simulink model "testGaitGeneration"  (R2016b)
settings: Solver=FixedStepAuto  StartTime=0.0  StopTime=20  FixedStep=0.001  RelTol=1e-3
undefined symbols (not defined in the file or in its folder): angleHip, angleKnee, GaitGenerator, lookUpTable, sitDownHip, sitDownKnee, standUpHip, standUpKnee, stateMachineHandler, walkRWHip, walkRWKnee
libraries: VariousLibrary x5, simulink x1
settings Model: DataDictionary=ModelDictionary.sldd  Creator=Taeke  LastModifiedBy=lucadelaat

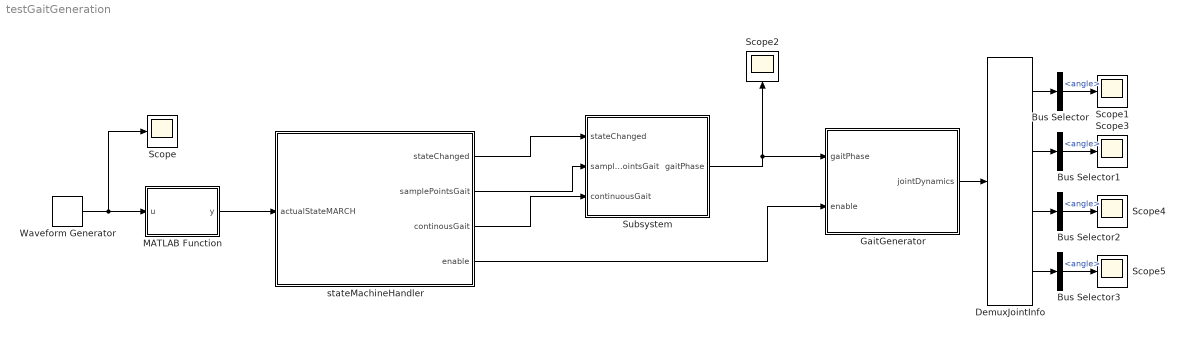
== system testGaitGeneration ==
  Bus Selector{,1..3} (4 alike) : BusSelector  OutputSignals=angle
  DemuxJointInfo : VariousLibrary/DemuxJointInfo
  GaitGenerator : Subsystem  AncestorBlock=lookUpTable/GaitGenerator
  MATLAB Function : MATLAB Function  TreatAsAtomicUnit=on
  Scope{,1..5} (6 alike) : Scope
  Subsystem : Subsystem  AncestorBlock=determinePhase/stateMachineHandler/Subsystem
  Waveform Generator : simulink/Sources/Waveform Generator  OutMin=[]  OutMax=[]  OutDataTypeStr=double  SelectedSignal=1  Signals=step(0,1,1)#step(10,0,1)  BlockNames=MultiportSwitch_2b879906c5d742a#MultiportSwitch_49a4cc9b4e66427  SampleTime=0.1
  stateMachineHandler : Subsystem  AncestorBlock=stateMachineHandler/stateMachineHandler
  wires:
  stateMachineHandler/1(stateChanged) -> Subsystem/1(stateChanged)
  stateMachineHandler/4(enable) -> GaitGenerator/2(enable)
  Subsystem/1(gaitPhase) -> GaitGenerator/1(gaitPhase), Scope2/1
  stateMachineHandler/2(samplePointsGait) -> Subsystem/2(samplePointsGait)
  GaitGenerator/1(jointDynamics) -> DemuxJointInfo/1
  DemuxJointInfo/4 -> Bus Selector3/1
  DemuxJointInfo/3 -> Bus Selector2/1
  DemuxJointInfo/2 -> Bus Selector1/1
  DemuxJointInfo/1 -> Bus Selector/1
  Bus Selector/1 -> Scope1/1  "<angle>"
  Bus Selector1/1 -> Scope3/1  "<angle>"
  Bus Selector2/1 -> Scope4/1  "<angle>"
  Bus Selector3/1 -> Scope5/1  "<angle>"
  stateMachineHandler/3(continousGait) -> Subsystem/3(continuousGait)
  MATLAB Function/1(y) -> stateMachineHandler/1(actualStateMARCH)
  Waveform Generator/1 -> Scope/1, MATLAB Function/1(u)

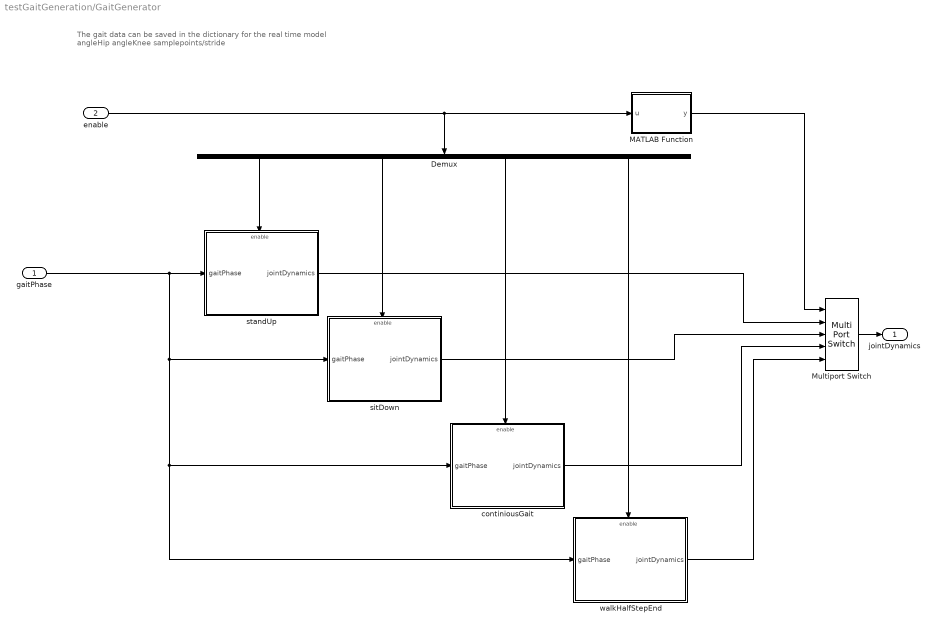
== system testGaitGeneration/GaitGenerator ==
  note: The gait data can be saved in the dictionary for the real time model
      | angleHip
      | angleKnee
      | samplepoints/stride
  gaitPhase : Inport
  enable : Inport  Port=2
  Demux : Demux
  MATLAB Function : MATLAB Function  TreatAsAtomicUnit=on
  Multiport Switch : MultiPortSwitch  Inputs=4  DataPortIndices={1,2,3,4}
  continiousGait : Subsystem
  "sitDown " : Subsystem
  standUp : Subsystem
  walkHalfStepEnd : Subsystem
  jointDynamics : Outport
  wires:
  Demux/1 -> standUp/Enable
  gaitPhase/1 -> "sitDown "/1(gaitPhase), walkHalfStepEnd/1(gaitPhase), continiousGait/1(gaitPhase), standUp/1(gaitPhase)
  continiousGait/1(jointDynamics) -> Multiport Switch/4
  Multiport Switch/1 -> jointDynamics/1
  walkHalfStepEnd/1(jointDynamics) -> Multiport Switch/5
  standUp/1(jointDynamics) -> Multiport Switch/2
  enable/1 -> MATLAB Function/1(u), Demux/1
  MATLAB Function/1(y) -> Multiport Switch/1
  Demux/2 -> "sitDown "/Enable
  Demux/3 -> continiousGait/Enable
  Demux/4 -> walkHalfStepEnd/Enable
  "sitDown "/1(jointDynamics) -> Multiport Switch/3

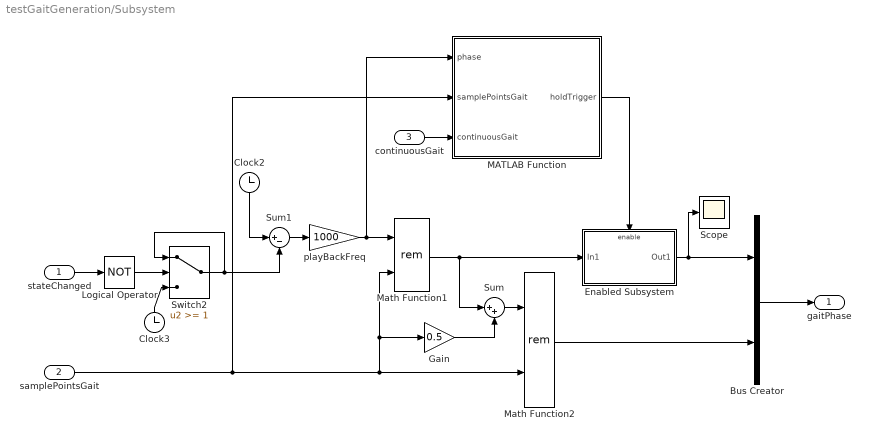
== system testGaitGeneration/Subsystem ==
  stateChanged : Inport
  samplePointsGait : Inport  Port=2
  continuousGait : Inport  Port=3
  Bus Creator : BusCreator  Inputs=2
  Clock2 : Clock
  Clock3 : Clock
      settings: Decimation=4
  Enabled Subsystem : Subsystem  TreatAsAtomicUnit=on
  Gain : Gain  Gain=0.5
  Logical Operator : Logic  Operator=NOT  AllPortsSameDT=off  OutDataTypeStr=boolean
  MATLAB Function : MATLAB Function  TreatAsAtomicUnit=on
  Math Function1 : Math  Operator=rem  SaturateOnIntegerOverflow=on
  Math Function2 : Math  Operator=rem  SaturateOnIntegerOverflow=on
  Scope : Scope
  Sum : Sum  Inputs=|++
  Sum1 : Sum  Inputs=|+-  SaturateOnIntegerOverflow=on  InputSameDT=on  OutDataTypeStr=Inherit: Same as first input
  Switch2 : Switch  Threshold=1  RndMeth=Zero
  playBackFreq : Gain  Gain=1000
  gaitPhase : Outport
  wires:
  playBackFreq/1 -> MATLAB Function/1(phase), Math Function1/1
  Sum1/1 -> playBackFreq/1
  Clock2/1 -> Sum1/1
  Clock3/1 -> Switch2/3
  Switch2/1 -> Switch2/1, Sum1/2
  Logical Operator/1 -> Switch2/2
  stateChanged/1 -> Logical Operator/1
  samplePointsGait/1 -> Gain/1, Math Function1/2, Math Function2/2, MATLAB Function/2(samplePointsGait)
  Math Function1/1 -> Sum/1, Enabled Subsystem/1(In1)
  Gain/1 -> Sum/2
  Sum/1 -> Math Function2/1
  Math Function2/1 -> Bus Creator/2
  Bus Creator/1 -> gaitPhase/1
  continuousGait/1 -> MATLAB Function/3(continuousGait)
  Enabled Subsystem/1(Out1) -> Scope/1, Bus Creator/1
  MATLAB Function/1(holdTrigger) -> Enabled Subsystem/Enable

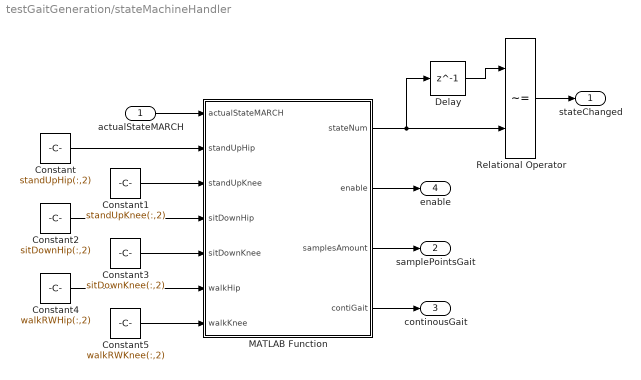
== system testGaitGeneration/stateMachineHandler ==
  actualStateMARCH : Inport
  Constant : Constant  Value=standUpHip(:,2)
  Constant1 : Constant  Value=standUpKnee(:,2)
  Constant2 : Constant  Value=sitDownHip(:,2)
  Constant3 : Constant  Value=sitDownKnee(:,2)
  Constant4 : Constant  Value=walkRWHip(:,2)
  Constant5 : Constant  Value=walkRWKnee(:,2)
  Delay : Delay  DelayLength=1  InitialCondition=0
  MATLAB Function : MATLAB Function  TreatAsAtomicUnit=on
  Relational Operator : RelationalOperator  Operator=~=  OutDataTypeStr=boolean  RndMeth=Simplest
  stateChanged : Outport  BusOutputAsStruct=on
  samplePointsGait : Outport  Port=2
  continousGait : Outport  Port=3
  enable : Outport  Port=4
  wires:
  Relational Operator/1 -> stateChanged/1
  Delay/1 -> Relational Operator/1
  actualStateMARCH/1 -> MATLAB Function/1(actualStateMARCH)
  MATLAB Function/3(samplesAmount) -> samplePointsGait/1
  MATLAB Function/2(enable) -> enable/1
  Constant/1 -> MATLAB Function/2(standUpHip)
  Constant1/1 -> MATLAB Function/3(standUpKnee)
  Constant2/1 -> MATLAB Function/4(sitDownHip)
  Constant3/1 -> MATLAB Function/5(sitDownKnee)
  Constant4/1 -> MATLAB Function/6(walkHip)
  Constant5/1 -> MATLAB Function/7(walkKnee)
  MATLAB Function/1(stateNum) -> Relational Operator/2, Delay/1
  MATLAB Function/4(contiGait) -> continousGait/1

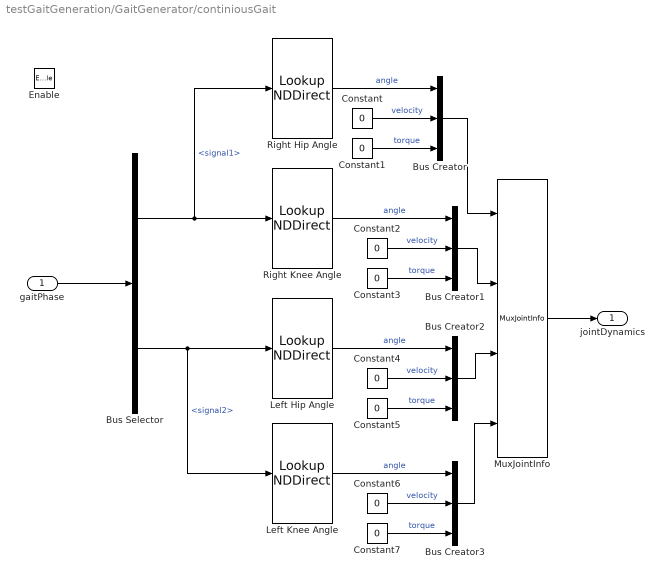
== system testGaitGeneration/GaitGenerator/continiousGait ==
  gaitPhase : Inport
  Enable : EnablePort
  Bus Creator{,1..3} (4 alike) : BusCreator  Inputs=3  OutDataTypeStr=Bus: JointDynamics  NonVirtualBus=on
  Bus Selector : BusSelector  OutputSignals=signal1,signal2
  Constant{,1..7} (8 alike) : Constant  Value=0
  Left Hip Angle : LookupNDDirect  NumberOfTableDimensions=1  Table=walkRWHip(:,2)
  Left Knee Angle : LookupNDDirect  NumberOfTableDimensions=1  Table=walkRWKnee(:,2)
  MuxJointInfo : VariousLibrary/MuxJointInfo
  Right Hip Angle : LookupNDDirect  NumberOfTableDimensions=1  Table=walkRWHip(:,2)
  Right Knee Angle : LookupNDDirect  NumberOfTableDimensions=1  Table=walkRWKnee(:,2)
  jointDynamics : Outport  OutDataTypeStr=Bus: JointDynamics
  wires:
  Right Hip Angle/1 -> Bus Creator/1  "angle"
  gaitPhase/1 -> Bus Selector/1
  Bus Selector/1 -> Right Hip Angle/1, Right Knee Angle/1  "<signal1>"
  Bus Selector/2 -> Left Knee Angle/1, Left Hip Angle/1  "<signal2>"
  MuxJointInfo/1 -> jointDynamics/1
  Constant/1 -> Bus Creator/2  "velocity"
  Constant1/1 -> Bus Creator/3  "torque"
  Bus Creator/1 -> MuxJointInfo/1
  Constant2/1 -> Bus Creator1/2  "velocity"
  Constant3/1 -> Bus Creator1/3  "torque"
  Right Knee Angle/1 -> Bus Creator1/1  "angle"
  Bus Creator1/1 -> MuxJointInfo/2
  Left Hip Angle/1 -> Bus Creator2/1  "angle"
  Constant4/1 -> Bus Creator2/2  "velocity"
  Constant5/1 -> Bus Creator2/3  "torque"
  Bus Creator2/1 -> MuxJointInfo/3
  Left Knee Angle/1 -> Bus Creator3/1  "angle"
  Constant6/1 -> Bus Creator3/2  "velocity"
  Constant7/1 -> Bus Creator3/3  "torque"
  Bus Creator3/1 -> MuxJointInfo/4

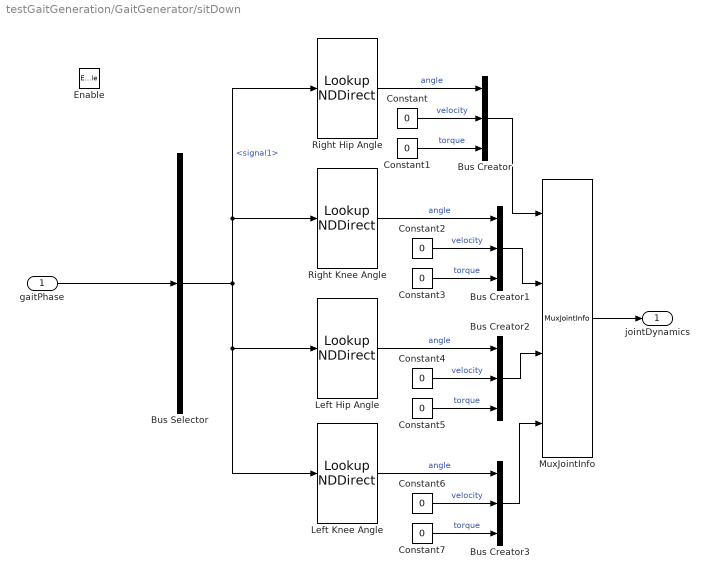
== system testGaitGeneration/GaitGenerator/sitDown  ==
  gaitPhase : Inport
  Enable : EnablePort
  Bus Creator{,1..3} (4 alike) : BusCreator  Inputs=3  OutDataTypeStr=Bus: JointDynamics  NonVirtualBus=on
  Bus Selector : BusSelector  OutputSignals=signal1
  Constant{,1..7} (8 alike) : Constant  Value=0
  Left Hip Angle : LookupNDDirect  NumberOfTableDimensions=1  Table=sitDownHip(:,2)
  Left Knee Angle : LookupNDDirect  NumberOfTableDimensions=1  Table=sitDownKnee(:,2)
  MuxJointInfo : VariousLibrary/MuxJointInfo
  Right Hip Angle : LookupNDDirect  NumberOfTableDimensions=1  Table=sitDownHip(:,2)
  Right Knee Angle : LookupNDDirect  NumberOfTableDimensions=1  Table=sitDownKnee(:,2)
  jointDynamics : Outport  OutDataTypeStr=Bus: JointDynamics
  wires:
  Right Hip Angle/1 -> Bus Creator/1  "angle"
  gaitPhase/1 -> Bus Selector/1
  Bus Selector/1 -> Left Knee Angle/1, Left Hip Angle/1, Right Hip Angle/1, Right Knee Angle/1  "<signal1>"
  MuxJointInfo/1 -> jointDynamics/1
  Constant/1 -> Bus Creator/2  "velocity"
  Constant1/1 -> Bus Creator/3  "torque"
  Bus Creator/1 -> MuxJointInfo/1
  Constant2/1 -> Bus Creator1/2  "velocity"
  Constant3/1 -> Bus Creator1/3  "torque"
  Right Knee Angle/1 -> Bus Creator1/1  "angle"
  Bus Creator1/1 -> MuxJointInfo/2
  Left Hip Angle/1 -> Bus Creator2/1  "angle"
  Constant4/1 -> Bus Creator2/2  "velocity"
  Constant5/1 -> Bus Creator2/3  "torque"
  Bus Creator2/1 -> MuxJointInfo/3
  Left Knee Angle/1 -> Bus Creator3/1  "angle"
  Constant6/1 -> Bus Creator3/2  "velocity"
  Constant7/1 -> Bus Creator3/3  "torque"
  Bus Creator3/1 -> MuxJointInfo/4

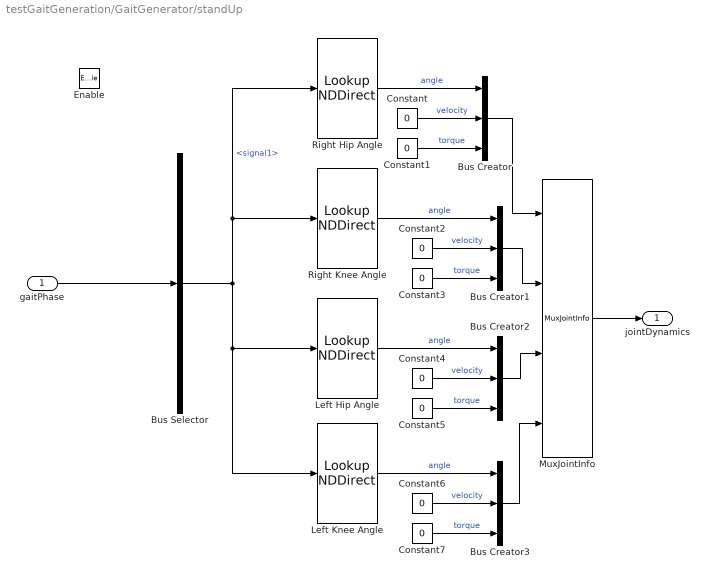
== system testGaitGeneration/GaitGenerator/standUp ==
  gaitPhase : Inport
  Enable : EnablePort
  Bus Creator{,1..3} (4 alike) : BusCreator  Inputs=3  OutDataTypeStr=Bus: JointDynamics  NonVirtualBus=on
  Bus Selector : BusSelector  OutputSignals=signal1
  Constant{,1..7} (8 alike) : Constant  Value=0
  Left Hip Angle : LookupNDDirect  NumberOfTableDimensions=1  Table=standUpHip(:,2)
  Left Knee Angle : LookupNDDirect  NumberOfTableDimensions=1  Table=standUpKnee(:,2)
  MuxJointInfo : VariousLibrary/MuxJointInfo
  Right Hip Angle : LookupNDDirect  NumberOfTableDimensions=1  Table=standUpHip(:,2)
  Right Knee Angle : LookupNDDirect  NumberOfTableDimensions=1  Table=standUpKnee(:,2)
  jointDynamics : Outport  OutDataTypeStr=Bus: JointDynamics
  wires:
  Right Hip Angle/1 -> Bus Creator/1  "angle"
  gaitPhase/1 -> Bus Selector/1
  Bus Selector/1 -> Left Knee Angle/1, Left Hip Angle/1, Right Hip Angle/1, Right Knee Angle/1  "<signal1>"
  MuxJointInfo/1 -> jointDynamics/1
  Constant/1 -> Bus Creator/2  "velocity"
  Constant1/1 -> Bus Creator/3  "torque"
  Bus Creator/1 -> MuxJointInfo/1
  Constant2/1 -> Bus Creator1/2  "velocity"
  Constant3/1 -> Bus Creator1/3  "torque"
  Right Knee Angle/1 -> Bus Creator1/1  "angle"
  Bus Creator1/1 -> MuxJointInfo/2
  Left Hip Angle/1 -> Bus Creator2/1  "angle"
  Constant4/1 -> Bus Creator2/2  "velocity"
  Constant5/1 -> Bus Creator2/3  "torque"
  Bus Creator2/1 -> MuxJointInfo/3
  Left Knee Angle/1 -> Bus Creator3/1  "angle"
  Constant6/1 -> Bus Creator3/2  "velocity"
  Constant7/1 -> Bus Creator3/3  "torque"
  Bus Creator3/1 -> MuxJointInfo/4

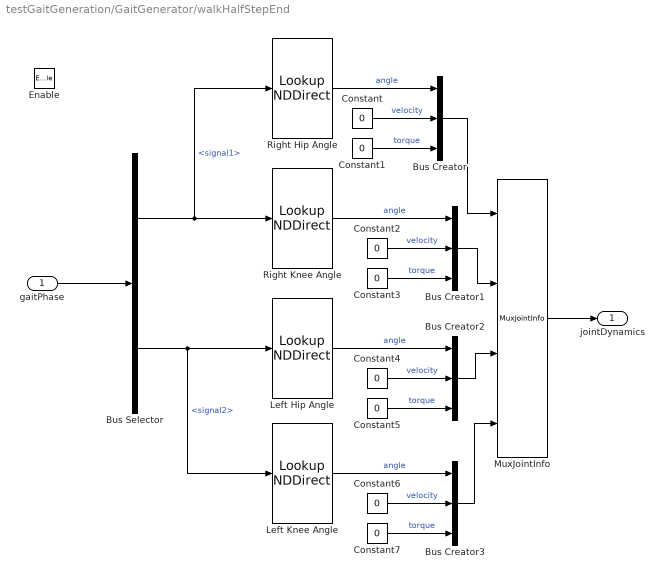
== system testGaitGeneration/GaitGenerator/walkHalfStepEnd ==
  gaitPhase : Inport
  Enable : EnablePort
  Bus Creator{,1..3} (4 alike) : BusCreator  Inputs=3  OutDataTypeStr=Bus: JointDynamics  NonVirtualBus=on
  Bus Selector : BusSelector  OutputSignals=signal1,signal2
  Constant{,1..7} (8 alike) : Constant  Value=0
  Left Hip Angle : LookupNDDirect  NumberOfTableDimensions=1  Table=angleHip
  Left Knee Angle : LookupNDDirect  NumberOfTableDimensions=1  Table=angleKnee
  MuxJointInfo : VariousLibrary/MuxJointInfo
  Right Hip Angle : LookupNDDirect  NumberOfTableDimensions=1  Table=angleHip
  Right Knee Angle : LookupNDDirect  NumberOfTableDimensions=1  Table=angleKnee
  jointDynamics : Outport  OutDataTypeStr=Bus: JointDynamics
  wires:
  Right Hip Angle/1 -> Bus Creator/1  "angle"
  gaitPhase/1 -> Bus Selector/1
  Bus Selector/1 -> Right Hip Angle/1, Right Knee Angle/1  "<signal1>"
  Bus Selector/2 -> Left Knee Angle/1, Left Hip Angle/1  "<signal2>"
  MuxJointInfo/1 -> jointDynamics/1
  Constant/1 -> Bus Creator/2  "velocity"
  Constant1/1 -> Bus Creator/3  "torque"
  Bus Creator/1 -> MuxJointInfo/1
  Constant2/1 -> Bus Creator1/2  "velocity"
  Constant3/1 -> Bus Creator1/3  "torque"
  Right Knee Angle/1 -> Bus Creator1/1  "angle"
  Bus Creator1/1 -> MuxJointInfo/2
  Left Hip Angle/1 -> Bus Creator2/1  "angle"
  Constant4/1 -> Bus Creator2/2  "velocity"
  Constant5/1 -> Bus Creator2/3  "torque"
  Bus Creator2/1 -> MuxJointInfo/3
  Left Knee Angle/1 -> Bus Creator3/1  "angle"
  Constant6/1 -> Bus Creator3/2  "velocity"
  Constant7/1 -> Bus Creator3/3  "torque"
  Bus Creator3/1 -> MuxJointInfo/4

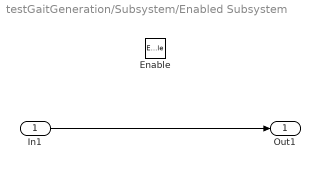
== system testGaitGeneration/Subsystem/Enabled Subsystem ==
  In1 : Inport
  Enable : EnablePort
  Out1 : Outport
  wires:
  In1/1 -> Out1/1

== matlab function testGaitGeneration/GaitGenerator/MATLAB Function ==
  data: u input; y output
function y = fcn(u)
y=0;
    if find(u,1)==1
        y=1;
    elseif find(u,1)==2
        y=2;
    elseif find(u,1)==3
        y=3;
    elseif find(u,1)==4
        y=4;
end
end

== matlab function testGaitGeneration/stateMachineHandler/MATLAB Function ==
  data: stateNum output; enable output; actualStateMARCH input; samplesAmount output; standUpHip input; standUpKnee input; sitDownHip input; sitDownKnee input; walkHip input; walkKnee input; contiGait output
function [stateNum, enable, samplesAmount, contiGait]= gaitSwitcher(actualStateMARCH, standUpHip, standUpKnee, sitDownHip, sitDownKnee, walkHip, walkKnee)
%#codegen

% This function is supposed to take a state and switch between controllers.
% Currently it directly routes the input argument as the index. In the
% future this can be something different so I have left it open for
% future modifications.

% The u vector represents the controllers. When the vector consists out of
% zeros it will not enable any controller. In the case that an index is set
% to a non zero value, the controller which belongs to that index will be
% enabled.

u=zeros(1,4);
stateNum=0;
samplesAmount=0;
contiGait=0;
        
switch actualStateMARCH
    case ExoskeletonState.STANDINGUP
    u(1) = 1;
    samplesAmount=length(standUpHip);
    stateNum=1;
    contiGait=0;
    
    case ExoskeletonState.SITTINGDOWN
    u(2) = 1;   
    samplesAmount=length(sitDownHip); 
    stateNum=2;
    contiGait=0;
    
    case ExoskeletonState.CONTINUOUSGAIT
    u(3) = 1;   
    samplesAmount=length(walkHip);  
    stateNum=3;
    contiGait=1;
end

enable = u;

== matlab function testGaitGeneration/Subsystem/MATLAB Function ==
  data: phase input; samplePointsGait input; continuousGait input; holdTrigger output
function holdTrigger = fcn(phase, samplePointsGait, continuousGait)
holdTrigger=1;
phase
samplePointsGait
if continuousGait==0 && phase>=samplePointsGait
    holdTrigger=0;
end

== matlab function testGaitGeneration/MATLAB Function ==
  data: u input; y output
function y = fcn(u)
if u==1
    y=ExoskeletonState.STANDINGUP
elseif u==2
    y=ExoskeletonState.SITTINGDOWN
elseif u==3
    y=ExoskeletonState.CONTINUOUSGAIT
else
    y=ExoskeletonState.HOLDSIT
end
